simulink model "EspacoDeEstados"  (R2021a)
settings: Solver=VariableStepAuto  StartTime=0.0  StopTime=10.0  RelTol=1e-3
undefined symbols (not defined in the file or in its folder): id, iq, Kdid, Kdidi, Kdiq, Kdiqi, Kdwi, Kqid, Kqidi, Kqiq, Kqiqi, Kqw, Kqwi, w
settings Model: Creator=migue  LastModifiedBy=migue

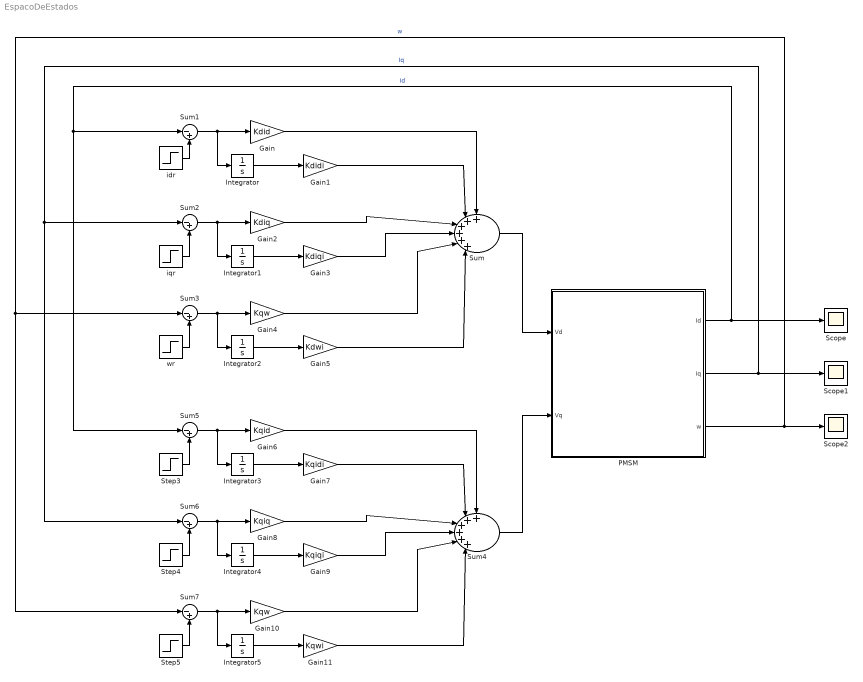
== system EspacoDeEstados ==
  Gain : Gain  Gain=Kdid
  Gain1 : Gain  Gain=Kdidi
  Gain10 : Gain  Gain=Kqw
  Gain11 : Gain  Gain=Kqwi
  Gain2 : Gain  Gain=Kdiq
  Gain3 : Gain  Gain=Kdiqi
  Gain4 : Gain  Gain=Kqw
  Gain5 : Gain  Gain=Kdwi
  Gain6 : Gain  Gain=Kqid
  Gain7 : Gain  Gain=Kqidi
  Gain8 : Gain  Gain=Kqiq
  Gain9 : Gain  Gain=Kqiqi
  Integrator{,1..5} (6 alike) : Integrator
  PMSM : Subsystem  mask{R=0.16, L=1.3e-4, N=10, J=1.8e-4, b=1e-5, lamb=0.06, Kt=0.095}
      mask prompts: R "Resitência (R)"; L "Indutância(L)"; N "Nº de par de polos(N)"; J "coeficiente(J)"; b "coeficiente(b)"; lamb "(lamb)"; Kt "(Kt)"
  Scope : Scope
  Scope1 : Scope
  Scope2 : Scope
  Step3 : Step  SampleTime=0
  Step4 : Step  SampleTime=0
  Step5 : Step  SampleTime=0
  Sum : Sum  Inputs=++++++|
  Sum{1..3,5..7} (6 alike) : Sum  Inputs=|-+
  Sum4 : Sum  Inputs=++++++|
  idr : Step  SampleTime=0
  iqr : Step  SampleTime=0
  wr : Step  SampleTime=0
  wires:
  Sum/1 -> PMSM/1(Vd)
  PMSM/1(Id) -> Scope/1, Sum1/1, Sum5/1  "Id"
  idr/1 -> Sum1/2
  Sum1/1 -> Integrator/1, Gain/1
  Gain/1 -> Sum/1
  Integrator/1 -> Gain1/1
  Gain1/1 -> Sum/2
  Integrator1/1 -> Gain3/1
  Sum2/1 -> Integrator1/1, Gain2/1
  iqr/1 -> Sum2/2
  PMSM/2(Iq) -> Sum2/1, Sum6/1, Scope1/1  "Iq"
  Gain2/1 -> Sum/3
  Gain3/1 -> Sum/4
  wr/1 -> Sum3/2
  Integrator2/1 -> Gain5/1
  Sum3/1 -> Integrator2/1, Gain4/1
  Gain4/1 -> Sum/5
  Gain5/1 -> Sum/6
  PMSM/3(w) -> Scope2/1, Sum3/1, Sum7/1  "w"
  Gain10/1 -> Sum4/5
  Gain7/1 -> Sum4/2
  Gain8/1 -> Sum4/3
  Integrator3/1 -> Gain7/1
  Gain6/1 -> Sum4/1
  Step3/1 -> Sum5/2
  Sum5/1 -> Integrator3/1, Gain6/1
  Integrator4/1 -> Gain9/1
  Sum7/1 -> Integrator5/1, Gain10/1
  Step5/1 -> Sum7/2
  Gain9/1 -> Sum4/4
  Step4/1 -> Sum6/2
  Integrator5/1 -> Gain11/1
  Sum6/1 -> Integrator4/1, Gain8/1
  Gain11/1 -> Sum4/6
  Sum4/1 -> PMSM/2(Vq)

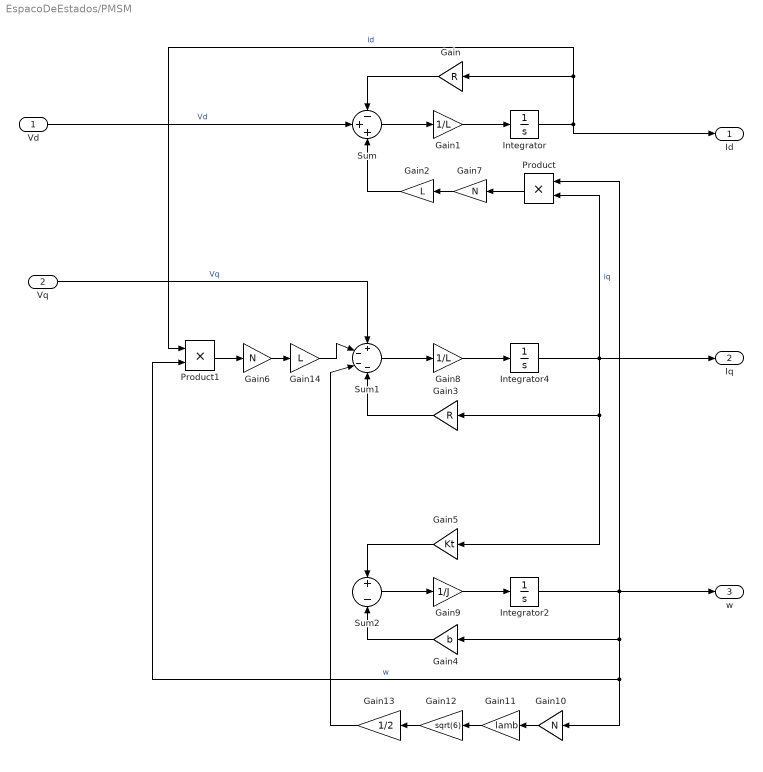
== system EspacoDeEstados/PMSM ==
  Vd : Inport
  Vq : Inport  Port=2
  Gain : Gain  Gain=R
  Gain1 : Gain  Gain=1/L
  Gain10 : Gain  Gain=N
  Gain11 : Gain  Gain=lamb
  Gain12 : Gain  Gain=sqrt(6)
  Gain13 : Gain  Gain=1/2
  Gain14 : Gain  Gain=L
  Gain2 : Gain  Gain=L
  Gain3 : Gain  Gain=R
  Gain4 : Gain  Gain=b
  Gain5 : Gain  Gain=Kt
  Gain6 : Gain  Gain=N
  Gain7 : Gain  Gain=N
  Gain8 : Gain  Gain=1/L
  Gain9 : Gain  Gain=1/J
  Integrator : Integrator  InitialCondition=id
  Integrator2 : Integrator  InitialCondition=w
  Integrator4 : Integrator  InitialCondition=iq
  Product : Product
  Product1 : Product
  Sum : Sum  Inputs=-++
  Sum1 : Sum  Inputs=+---
  Sum2 : Sum  Inputs=+-
  Id : Outport
  Iq : Outport  Port=2
  w : Outport  Port=3
  wires:
  Integrator4/1 -> Iq/1, Product/2, Gain3/1, Gain5/1  "iq"
  Integrator/1 -> Gain/1, Product1/1, Id/1  "id"
  Gain8/1 -> Integrator4/1
  Sum1/1 -> Gain8/1
  Product1/1 -> Gain6/1
  Gain/1 -> Sum/1
  Sum2/1 -> Gain9/1
  Integrator2/1 -> w/1, Product/1, Gain10/1, Product1/2, Gain4/1  "w"
  Gain5/1 -> Sum2/1
  Vd/1 -> Sum/2  "Vd"
  Gain9/1 -> Integrator2/1
  Gain1/1 -> Integrator/1
  Sum/1 -> Gain1/1
  Gain4/1 -> Sum2/2
  Gain3/1 -> Sum1/4
  Gain11/1 -> Gain12/1
  Gain10/1 -> Gain11/1
  Product/1 -> Gain7/1
  Vq/1 -> Sum1/1  "Vq"
  Gain12/1 -> Gain13/1
  Gain13/1 -> Sum1/3
  Gain6/1 -> Gain14/1
  Gain7/1 -> Gain2/1
  Gain2/1 -> Sum/3
  Gain14/1 -> Sum1/2
